simulink model "SimConnectToolbox_Test"  (R2021b)
settings: Solver=FixedStepDiscrete  StartTime=0.0  StopTime=inf  FixedStep=0.03  RelTol=1e-3
undefined symbols (not defined in the file or in its folder): aux
libraries: SimConnectToolbox x2
settings Model: Creator=Andreas  LastModifiedBy=ccortes9
settings SolverCC: AlgebraicLoopSolver=TrustRegion
settings DebuggingCC: InheritedTsInSrcMsg=none  SFMachineParentedDataDiag=warning

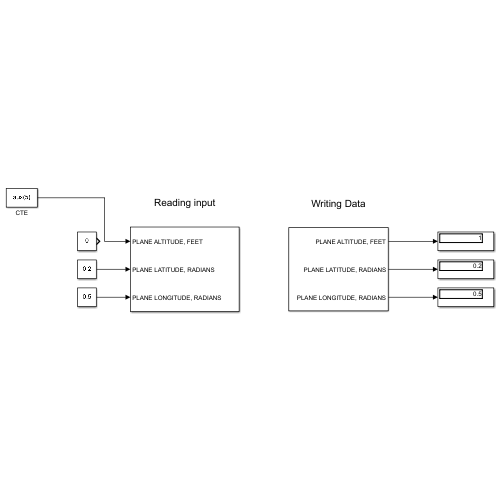
[thumbnail: Simulink's stored preview of the top-level diagram]
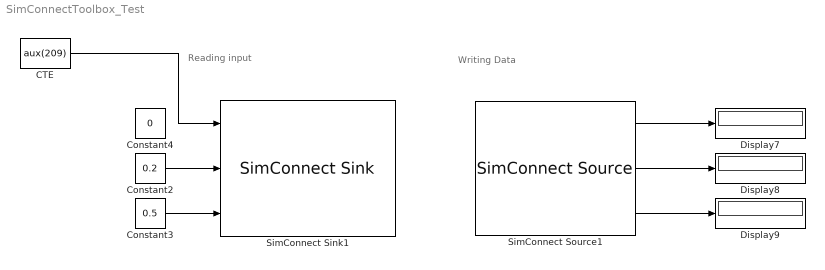
== system SimConnectToolbox_Test ==
  note: Reading input
  note: Writing Data
  CTE : Constant  Value=aux(209)  SampleTime=0.03
  Constant2 : Constant  Value=0.2  SampleTime=0.03
  Constant3 : Constant  Value=0.5  SampleTime=0.03
  Constant4 : Constant  Value=0  SampleTime=0.03
  Display7 : Display
  Display8 : Display
  Display9 : Display
  SimConnect Sink1 : SimConnectToolbox/SimConnect Sink  configurationIndex=0  connectionName=SimConnectSink  variables=|
      | PLANE ALTITUDE, FEET;
      | PLANE LATITUDE, RADIANS;
      | PLANE LONGITUDE, RADIANS;
      settings: SourceProductName=SimConnect Toolbox
      mask Display:
      | % This is a new mask on top of the base mask.
      | % Use "View base mask" link below to see the base mask.
      | %port_label('input', 1, 'Rudder Trim', 'texmode', 'on')
      | port_label('input', 1, 'PLANE ALTITUDE, FEET', 'texmode', 'on')
      | port_label('input', 2, 'PLANE LATITUDE, RADIANS', 'texmode', 'on')
      | port_label('input', 3, 'PLANE LONGITUDE, RADIANS', 'texmode', 'on')
  SimConnect Source1 : SimConnectToolbox/SimConnect Source  configurationIndex=0  connectionName=SimConnectSource  variables=|
      | PLANE ALTITUDE, FEET;
      | PLANE LATITUDE, RADIANS;
      | PLANE LONGITUDE, RADIANS;
      settings: SourceProductName=SimConnect Toolbox
      mask Display:
      | % This is a new mask on top of the base mask.
      | % Use "View base mask" link below to see the base mask.
      | % port_label('output', 1, 'g', 'texmode', 'on')
      | port_label('output', 1, 'PLANE ALTITUDE, FEET', 'texmode', 'on')
      | port_label('output', 2, 'PLANE LATITUDE, RADIANS', 'texmode', 'on')
      | port_label('output', 3, 'PLANE LONGITUDE, RADIANS', 'texmode', 'on')
  wires:
  SimConnect Source1/1 -> Display7/1
  SimConnect Source1/2 -> Display8/1
  SimConnect Source1/3 -> Display9/1
  Constant2/1 -> SimConnect Sink1/2
  Constant3/1 -> SimConnect Sink1/3
  CTE/1 -> SimConnect Sink1/1
